simulink model "ICAES"  (R2025b)
settings: Solver=FixedStepAuto  StartTime=0.0  StopTime=stopt  FixedStep=deltat  MaxStep=0.05  RelTol=1e-3
InitFcn:
  | clear all;
  | close all;
  | clc;
  | 
  | % add the data and script directories
  | addpath('data','scripts');
  | 
  | % load the constants (units)
  | constants;
  | 
  | % load the simulation parameters
  | preprocessing;
StopFcn:
  | postprocessing;
values from neighbouring files (symbols this model uses):
  A_tes = 2500 * unit("m^2")    [preprocessing.m]
  c_p = 1005    [icaes_parameter_sweep.m]    (also in preprocessing.m = 1005 * unit("J") / (unit("kg") * unit("K")))
  c_tes = 4184    [icaes_parameter_sweep.m]    (also in preprocessing.m = 4184 * unit("J") / (unit("kg") * unit("K")))
  eta_comp = 0.833    [icaes_parameter_sweep.m]    (also in preprocessing.m)
  eta_exp = 0.85    [icaes_parameter_sweep.m]    (also in preprocessing.m)
  eta_tran = 0.97    [icaes_parameter_sweep.m]    (also in preprocessing.m)
  m_tes = m_tes_range(im)    [icaes_parameter_sweep.m]    (also in preprocessing.m = 20000000 * unit("kg"))
  n_poly = 1.1    [icaes_parameter_sweep.m]    (also in preprocessing.m)
  p_amb = 101325    [icaes_parameter_sweep.m]    (also in preprocessing.m = 101325 * unit("Pa"))
  P_limit = 300e6    (= 300000000)    [icaes_parameter_sweep.m]    (also in preprocessing.m = 300 * unit("MW"))
  p_store_initial = 40 * unit("bar")    [preprocessing.m]
  p_store_max = 100e5    (= 10000000)    [icaes_parameter_sweep.m]    (also in preprocessing.m = 80 * unit("bar"))
  R_air = 287.05    [icaes_parameter_sweep.m]    (also in preprocessing.m = 287.05 * unit("J") / (unit("kg") * unit("K")))
  T_amb = 300    [icaes_parameter_sweep.m]    (also in preprocessing.m = 300 * unit("K"))
  T_tes_initial = T_amb    [preprocessing.m]
  T_tes_max = 373 * unit("K")    [preprocessing.m]
  U_tes = 2.0    (= 2)    [preprocessing.m]
  V_cavern = V_cav_range(iv)    [icaes_parameter_sweep.m]    (also in preprocessing.m = 5000000 * unit("m^3"))
settings Model: Creator=joche  LastModifiedBy=ASUS
settings DataIOCC: SaveFormat=Array  SaveOutput=off  ReturnWorkspaceOutputs=off
settings OptimizationCC: ReuseModelBlockBuffer=off
settings ModelReferenceCC: EnableRefExpFcnMdlSchedulingChecks=on
settings RTWCC: GPUComputeCapability=3.5
settings SimscapeCC: SimscapeLogDecimation=1  SimscapeLogDataHistory=5000

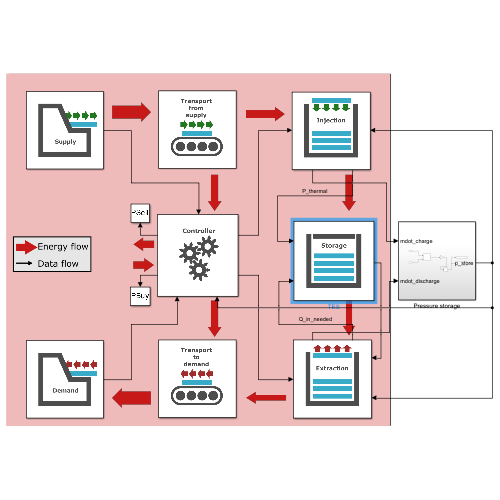
[thumbnail: Simulink's stored preview of the top-level diagram]
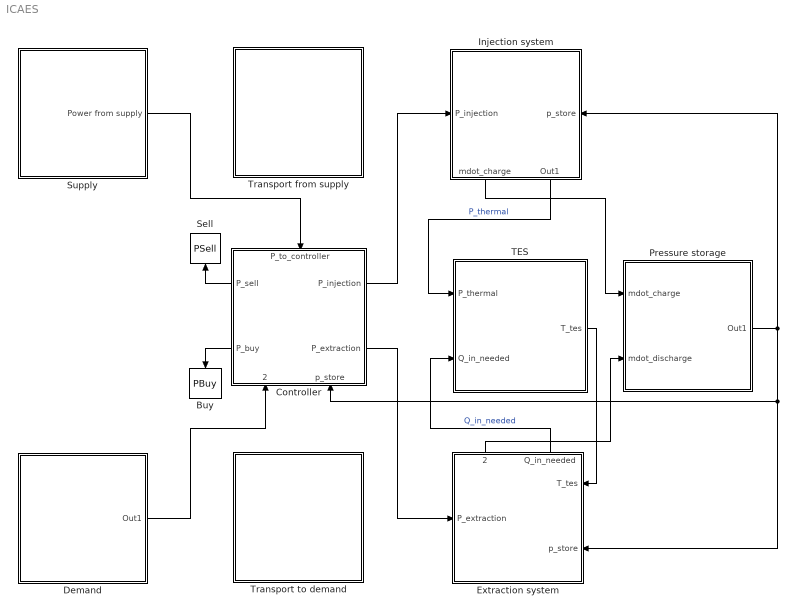
== system ICAES ==
  Buy : ToWorkspace  VariableName=PBuy  SampleTime=-1
  Controller : Subsystem
      settings: PortSchema="{\"entries\":[{\"content\":{\"sides\":[{\"content\":{\"connectorIds\":[\"Out3\",\"Out4\"]},\"type\":\"ConnectorPlacement.EquallySpacedRectSide\",\"uuid\":\"4daf33ce-c96a-4783-b5c4-228eed953e01\"},{\"content\":{\"connectorIds\":[\"Out1\",\"Out2\"],\"side\":\"RIGHT\"},\"type\":\"ConnectorPlacement.EquallySpacedRectSide\",\"uuid\":\"e9942e50-8467-4af8-b79b-80636cbc76e5\"},{\"content\":{\"connectorIds\":[\"In1\"],\"side\":\"TOP\"},\"type\":\"ConnectorPlacement.EquallySpacedRectSide\",\"uuid\":\"f315e931-d69b-4751-b712-f89c6c81baeb\"},{\"content\":{\"connectorIds\":[\"In2\",\"In3\"],\"side\":\"BOTTOM\"},\"type\":\"ConnectorPlacement.EquallySpacedRectSide\",\"uuid\":\"44715ee6-5cd5-4669-bcb9-5ed7c869bdb3\"}]},\"type\":\"ConnectorPlacement.EquallySpacedConnector\",\"uuid\":\"fff48899-944b-4064-b7d7-ecc12144fb48\"}],\"packageUris\":[\"http://schema.mathworks.com/mf0/Connector/R2020b\"],\"version\":\"1.0\"}"
      mask Display: image('$imagefile'); % Use "Edit Image" on toolstrip to change.
  Demand : Subsystem
      mask Display: image('$imagefile'); % Use "Edit Image" on toolstrip to change.
  Extraction system : Subsystem
      settings: PortSchema="{\"entries\":[{\"content\":{\"sides\":[{\"content\":{\"connectorIds\":[\"In1\",\"In2\"]},\"type\":\"ConnectorPlacement.EquallySpacedRectSide\",\"uuid\":\"05c5933d-55fc-4e06-853f-fc26d42905f9\"},{\"content\":{\"connectorIds\":[\"In3\"],\"side\":\"RIGHT\"},\"type\":\"ConnectorPlacement.EquallySpacedRectSide\",\"uuid\":\"327426c5-31d5-498b-a2bd-83e49353408c\"},{\"content\":{\"side\":\"TOP\"},\"type\":\"ConnectorPlacement.EquallySpacedRectSide\",\"uuid\":\"55306cf3-a3de-4385-a5ae-b8600ecdd5a2\"},{\"content\":{\"connectorIds\":[\"Out1\",\"Out2\"],\"side\":\"BOTTOM\"},\"type\":\"ConnectorPlacement.EquallySpacedRectSide\",\"uuid\":\"08fcc9c3-40d3-4ac6-b914-dfeef6039ffb\"}]},\"type\":\"ConnectorPlacement.EquallySpacedConnector\",\"uuid\":\"cb35d5ba-e8c6-462c-b7b2-fe8356d4b0a1\"}],\"packageUris\":[\"http://schema.mathworks.com/mf0/Connector/R2020b\"],\"version\":\"1.0\"}"
      mask Display: image('$imagefile'); % Use "Edit Image" on toolstrip to change.
  Injection system : Subsystem
      settings: PortSchema="{\"entries\":[{\"content\":{\"sides\":[{\"content\":{\"connectorIds\":[\"In1\"]},\"type\":\"ConnectorPlacement.EquallySpacedRectSide\",\"uuid\":\"05c5933d-55fc-4e06-853f-fc26d42905f9\"},{\"content\":{\"connectorIds\":[\"In2\"],\"side\":\"RIGHT\"},\"type\":\"ConnectorPlacement.EquallySpacedRectSide\",\"uuid\":\"327426c5-31d5-498b-a2bd-83e49353408c\"},{\"content\":{\"connectorIds\":[\"Out1\",\"Out2\"],\"side\":\"TOP\"},\"type\":\"ConnectorPlacement.EquallySpacedRectSide\",\"uuid\":\"55306cf3-a3de-4385-a5ae-b8600ecdd5a2\"},{\"content\":{\"side\":\"BOTTOM\"},\"type\":\"ConnectorPlacement.EquallySpacedRectSide\",\"uuid\":\"08fcc9c3-40d3-4ac6-b914-dfeef6039ffb\"}]},\"type\":\"ConnectorPlacement.EquallySpacedConnector\",\"uuid\":\"cb35d5ba-e8c6-462c-b7b2-fe8356d4b0a1\"}],\"packageUris\":[\"http://schema.mathworks.com/mf0/Connector/R2020b\"],\"version\":\"1.0\"}"
      mask Display: image('$imagefile'); % Use "Edit Image" on toolstrip to change.
  Pressure storage : Subsystem
  Sell : ToWorkspace  VariableName=PSell  SampleTime=-1
  Supply : Subsystem
      mask Display: image('$imagefile'); % Use "Edit Image" on toolstrip to change.
  TES : Subsystem
      mask Display: image('$imagefile'); % Use "Edit Image" on toolstrip to change.
  Transport from supply : Subsystem
      mask Display: image('$imagefile'); % Use "Edit Image" on toolstrip to change.
  Transport to demand : Subsystem
      mask Display: image('$imagefile'); % Use "Edit Image" on toolstrip to change.
  wires:
  Controller/3(P_sell) -> Sell/1
  Controller/2(P_extraction) -> Extraction system/3(P_extraction)
  Controller/1(P_injection) -> Injection system/2(P_injection)
  Controller/4(P_buy) -> Buy/1
  Pressure storage/1(Out1) -> Injection system/1(p_store), Controller/3(p_store), Extraction system/1(p_store)
  Injection system/1(Out1) -> TES/1(P_thermal)  "P_thermal"
  Extraction system/1(Q_in_needed) -> TES/2(Q_in_needed)  "Q_in_needed"
  TES/1(T_tes) -> Extraction system/2(T_tes)
  Supply/1(Power from supply) -> Controller/1(P_to_controller)
  Demand/1(Out1) -> Controller/2(P_from_controller)
  Extraction system/2(mdot_discharge) -> Pressure storage/2(mdot_discharge)
  Injection system/2(mdot_charge) -> Pressure storage/1(mdot_charge)

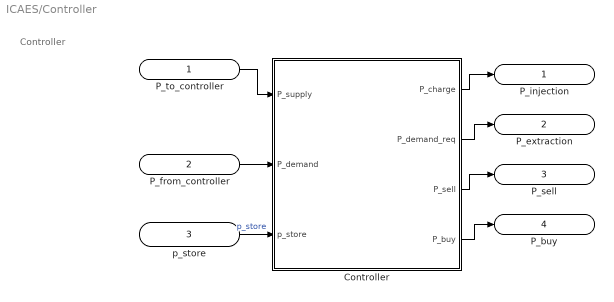
== system ICAES/Controller ==
  note: Controller
  P_to_controller : Inport
  P_from_controller : Inport  Port=2
  p_store : Inport  Port=3
  Controller : MATLAB Function  TreatAsAtomicUnit=on
  P_injection : Outport
  P_extraction : Outport  Port=2
  P_sell : Outport  Port=3
  P_buy : Outport  Port=4
  wires:
  P_from_controller/1 -> Controller/2(P_demand)
  Controller/2(P_demand_req) -> P_extraction/1
  Controller/3(P_sell) -> P_sell/1
  Controller/4(P_buy) -> P_buy/1
  P_to_controller/1 -> Controller/1(P_supply)
  Controller/1(P_charge) -> P_injection/1
  p_store/1 -> Controller/3(p_store)  "p_store"

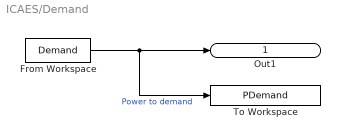
== system ICAES/Demand ==
  From Workspace : FromWorkspace  VariableName=Demand  OutputAfterFinalValue=Setting to zero
  To Workspace : ToWorkspace  VariableName=PDemand  SampleTime=-1
  Out1 : Outport
  wires:
  From Workspace/1 -> To Workspace/1, Out1/1  "Power to demand"

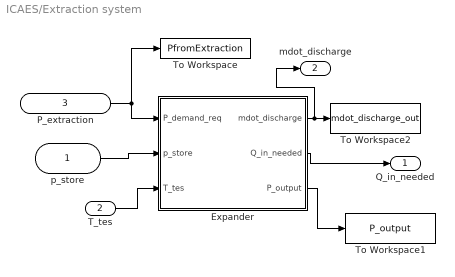
== system ICAES/Extraction system ==
  p_store : Inport
  T_tes : Inport  Port=2
  P_extraction : Inport  Port=3
  Expander : MATLAB Function  TreatAsAtomicUnit=on
  To Workspace : ToWorkspace  VariableName=PfromExtraction  SampleTime=-1
  To Workspace1 : ToWorkspace  VariableName=P_output  SampleTime=-1
  To Workspace2 : ToWorkspace  VariableName=mdot_discharge_out  SampleTime=-1
  Q_in_needed : Outport
  mdot_discharge : Outport  Port=2
  wires:
  P_extraction/1 -> To Workspace/1, Expander/1(P_demand_req)
  p_store/1 -> Expander/2(p_store)
  Expander/3(P_output) -> To Workspace1/1
  Expander/2(Q_in_needed) -> Q_in_needed/1
  T_tes/1 -> Expander/3(T_tes)
  Expander/1(mdot_discharge) -> mdot_discharge/1, To Workspace2/1

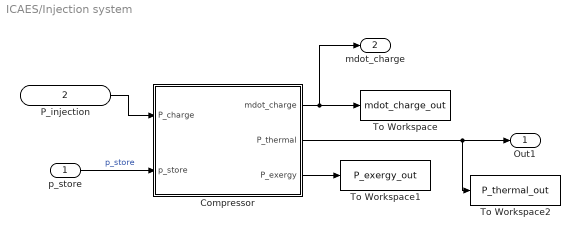
== system ICAES/Injection system ==
  p_store : Inport
  P_injection : Inport  Port=2
  Compressor : MATLAB Function  TreatAsAtomicUnit=on
  To Workspace : ToWorkspace  VariableName=mdot_charge_out  SampleTime=-1
  To Workspace1 : ToWorkspace  VariableName=P_exergy_out  SampleTime=-1
  To Workspace2 : ToWorkspace  VariableName=P_thermal_out  SampleTime=-1
  Out1 : Outport
  mdot_charge : Outport  Port=2
  wires:
  P_injection/1 -> Compressor/1(P_charge)
  p_store/1 -> Compressor/2(p_store)  "p_store"
  Compressor/2(P_thermal) -> To Workspace2/1, Out1/1
  Compressor/3(P_exergy) -> To Workspace1/1
  Compressor/1(mdot_charge) -> mdot_charge/1, To Workspace/1

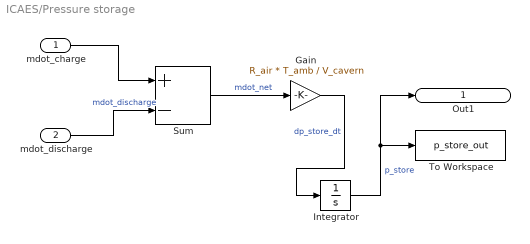
== system ICAES/Pressure storage ==
  mdot_charge : Inport
  mdot_discharge : Inport  Port=2
  Gain : Gain  Gain=R_air * T_amb / V_cavern
  Integrator : Integrator  InitialCondition=p_store_initial
  Sum : Sum  Inputs=+-
  To Workspace : ToWorkspace  VariableName=p_store_out  SampleTime=-1
  Out1 : Outport
  wires:
  Gain/1 -> Integrator/1  "dp_store_dt"
  mdot_discharge/1 -> Sum/2  "mdot_discharge"
  Integrator/1 -> Out1/1, To Workspace/1  "p_store"
  mdot_charge/1 -> Sum/1
  Sum/1 -> Gain/1  "mdot_net"

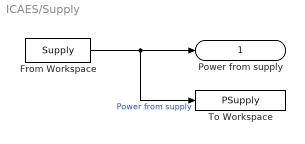
== system ICAES/Supply ==
  From Workspace : FromWorkspace  VariableName=Supply  OutputAfterFinalValue=Setting to zero
  To Workspace : ToWorkspace  VariableName=PSupply  SampleTime=-1
  Power from supply : Outport
  wires:
  From Workspace/1 -> To Workspace/1, Power from supply/1  "Power from supply"

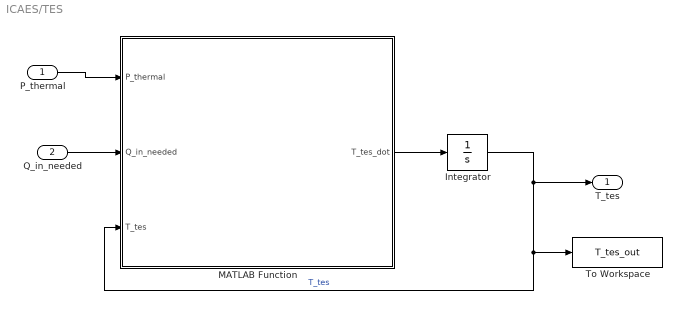
== system ICAES/TES ==
  P_thermal : Inport
  Q_in_needed : Inport  Port=2
  Integrator : Integrator  InitialCondition=T_tes_initial  LimitOutput=on  UpperSaturationLimit=T_tes_max  LowerSaturationLimit=T_amb
  MATLAB Function : MATLAB Function  TreatAsAtomicUnit=on
  To Workspace : ToWorkspace  VariableName=T_tes_out  SampleTime=-1
  T_tes : Outport
  wires:
  P_thermal/1 -> MATLAB Function/1(P_thermal)
  Q_in_needed/1 -> MATLAB Function/2(Q_in_needed)
  MATLAB Function/1(T_tes_dot) -> Integrator/1
  Integrator/1 -> T_tes/1, To Workspace/1, MATLAB Function/3(T_tes)  "T_tes"

== system ICAES/Transport from supply ==

== system ICAES/Transport to demand ==

== matlab function ICAES/Injection system/Compressor ==
  data: P_charge input; mdot_charge output; p_store input; P_thermal output; P_exergy output; eta_comp parameter; n_poly parameter; R_air parameter; c_p parameter; T_amb parameter; p_amb parameter
function [mdot_charge, P_thermal, P_exergy] = compressor( ...
    P_charge, p_store, ...
    eta_comp, n_poly, R_air, c_p, T_amb, p_amb)
%COMPRESSOR  Polytropic compression.
%   Converts electrical power into thermal energy (→TES) and
%   pressure exergy (→Cavern) via mass flow of compressed air.
%
%   Equations from model: (2.8), (2.9), (2.10), (2.11)

    mdot_charge = 0;
    P_thermal = 0;
    P_exergy = 0;

    if P_charge <= 0
        return;
    end

    % Pressure ratio
    ratio = p_store / p_amb;
    if ratio <= 1
        ratio = 1.001;  % Guard: cavern at ambient
    end

    % Polytropic work factor [J/kg]
    poly_factor = (n_poly/(n_poly-1)) * R_air * T_amb * (ratio^((n_poly-1)/n_poly) - 1);

    % Mass flow rate [kg/s]   — Eq. 2.9
    mdot_charge = P_charge / (eta_comp * poly_factor);

    % Compressor outlet temperature [K]
    T_out = T_amb * ratio^((n_poly-1)/n_poly);

    % Thermal power to TES [W]  — Eq. 2.10
    P_thermal = P_charge - mdot_charge * c_p * (T_out - T_amb);
    if P_thermal < 0
        P_thermal = 0;  % Guard
    end

    % Pressure exergy rate [W]  — Eq. 2.11
    P_exergy = mdot_charge * R_air * T_amb * log(ratio);
end

== matlab function ICAES/Controller/Controller ==
  data: P_charge output; P_demand_req output; P_sell output; P_buy output; P_supply input; P_demand input; p_store input; eta_tran parameter; P_limit parameter; p_store_max parameter; p_amb parameter
function [P_charge, P_demand_req, P_sell, P_buy] = controller( ...
    P_supply, P_demand, p_store, ...
    eta_tran, P_limit, p_store_max, p_amb)
%CONTROLLER  Determines charging/discharging mode based on P_net.
%   P_net >= 0  →  charge (compress air)
%   P_net <  0  →  discharge (expand air)

    P_net = P_supply - P_demand;

    % Default outputs
    P_charge = 0;
    P_demand_req = 0;
    P_sell = 0;
    P_buy = 0;

    if P_net >= 0
        % === CHARGING MODE ===
        P_available = min(P_net, P_limit);
        P_charge = eta_tran * P_available;
        P_sell = (P_net - P_available);       % Excess beyond P_limit

        % Stop charging if cavern full
        if p_store >= p_store_max
            P_sell = P_sell + P_charge;
            P_charge = 0;
        end
    else
        % === DISCHARGING MODE ===
        P_demand_req = -P_net;                % Positive value

        % Stop discharging if cavern nearly empty
        if p_store <= p_amb * 1.05
            P_buy = P_demand_req;
            P_demand_req = 0;
        end
    end
end

== matlab function ICAES/Extraction system/Expander ==
  data: P_demand_req input; mdot_discharge output; p_store input; Q_in_needed output; T_tes input; P_output output; eta_exp parameter; eta_tran parameter; n_poly parameter; R_air parameter; c_p parameter; p_amb parameter
function [mdot_discharge, Q_in_needed, P_output] = expander( ...
    P_demand_req, p_store, T_tes, ...
    eta_exp, eta_tran, n_poly, R_air, c_p, p_amb)
%EXPANDER  Polytropic expansion.
%   Extracts energy from cavern pressure + TES heat → electricity.
%
%   Equations from model: (2.15), (2.18), (2.19)

    mdot_discharge = 0;
    Q_in_needed = 0;
    P_output = 0;

    if P_demand_req <= 0
        return;
    end

    % Required discharge power before transmission loss
    P_discharge = P_demand_req / eta_tran;

    % Pressure ratio (expansion direction)
    ratio = p_amb / p_store;
    if ratio >= 1
        return;  % No pressure difference → cannot expand
    end

    % Expansion inlet temperature = TES temperature
    T_in = T_tes;

    % Polytropic expansion factor [J/kg]  — Eq. 2.15
    poly_factor = (n_poly/(n_poly-1)) * R_air * T_in * (1 - ratio^((n_poly-1)/n_poly));

    if poly_factor <= 0
        return;  % Guard
    end

    % Mass flow rate [kg/s]
    mdot_discharge = P_discharge / (eta_exp * poly_factor);

    % Expander outlet temperature [K]
    T_out = T_in * ratio^((n_poly-1)/n_poly);

    % Thermal power drawn from TES [W]  — Eq. 2.18
    Q_in_needed = P_discharge / eta_exp - mdot_discharge * c_p * (T_in - T_out);
    if Q_in_needed < 0
        Q_in_needed = 0;
    end

    % Power delivered to grid [W]  — Eq. 2.19
    P_output = eta_tran * P_discharge;
end

== matlab function ICAES/TES/MATLAB Function ==
  data: P_thermal input; T_tes_dot output; Q_in_needed input; T_tes input; T_amb parameter; U_tes parameter; A_tes parameter; m_tes parameter; c_tes parameter
function T_tes_dot = tes_dynamics(P_thermal, Q_in_needed, T_tes, ...
    T_amb, U_tes, A_tes, m_tes, c_tes)
%TES_DYNAMICS  Thermal energy storage temperature ODE.
%   Eq. 2.13: m·c · dT/dt = P_in − Q_out − Q_loss
    % Heat loss to environment
    Q_loss = U_tes * A_tes * (T_tes - T_amb);
    % Temperature rate of change
    T_tes_dot = (P_thermal - Q_in_needed - Q_loss) / (m_tes * c_tes);
end
